simulink model "ABS_CAN_MBD"  (R2024b)
settings: Solver=FixedStepAuto  StartTime=0.0  StopTime=15  FixedStep=0.01  RelTol=1e-3
undefined symbols (not defined in the file): canChannel, g, I, m, R, v0
libraries: canlib x3, canmsglib x2
settings Model: Creator=Stephen Kingston  LastModifiedBy=chinmay
settings SolverCC: AlgebraicLoopSolver=TrustRegion
settings DebuggingCC: UnconnectedInputMsg=warning  UnconnectedOutputMsg=warning  UnconnectedLineMsg=warning
settings ModelReferenceCC: EnableRefExpFcnMdlSchedulingChecks=on
settings SFSimCC: CustomCodeUndefinedFunction=UseInterfaceOnly
settings RTWCC: GPUComputeCapability=3.5

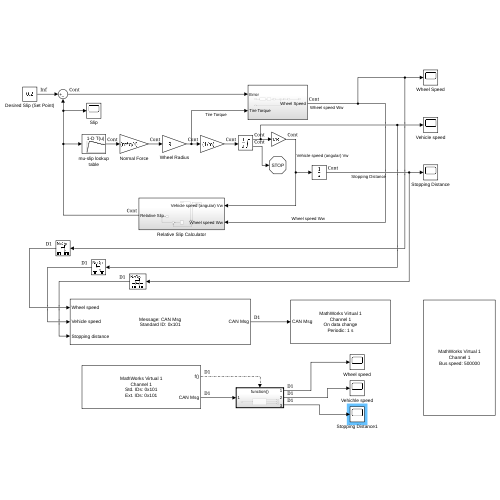
[thumbnail: Simulink's stored preview of the top-level diagram]
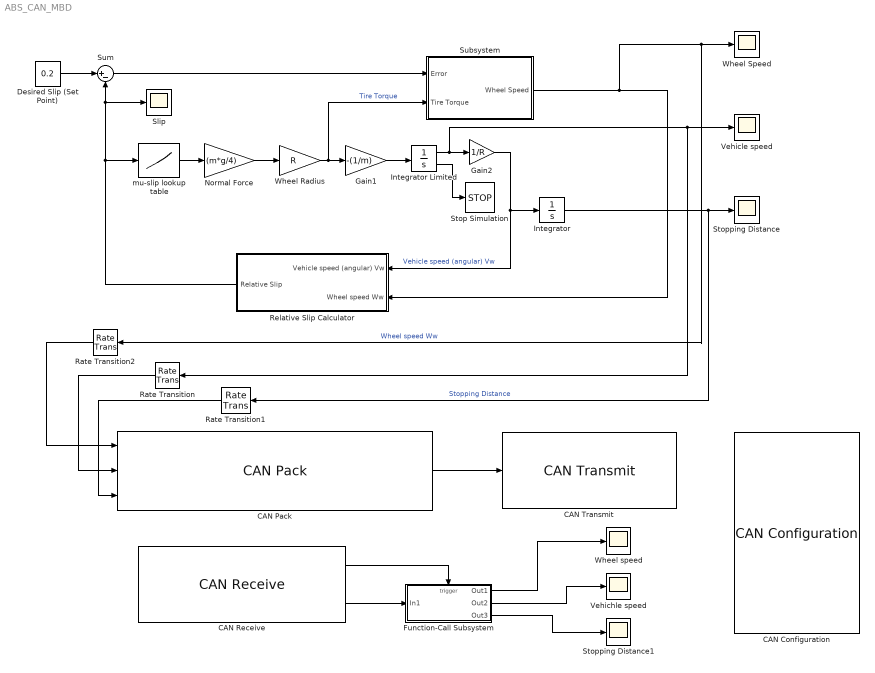
== system ABS_CAN_MBD ==
  CAN Configuration : canlib/CAN Configuration  BlockHandle=495.0005  Device=MathWorks Virtual 1 (Channel 1)  DeviceMenu=MathWorks Virtual 1 (Channel 1)  ObjConstructor=canChannel('MathWorks', 'Virtual 1', 1)  BusSpeed=500000  EnableBitParameters=off  AckMode=Normal
  CAN Pack : canmsglib/CAN Pack  MsgList=(none)  MsgName=CAN Msg  MsgIDType=Standard (11-bit identifier)  MsgIdentifier=0x101  CANIDInput=off  MsgLength=8  Remote=off  ApplyMinMax=off  BusOutput=off  SignalInfo={ 'Wheel speed', '0', '16', 'LE', 'unsigned', 'Standard', '0', '1', '0', '-Inf', 'Inf'; 'Vehicle speed', '16', '16', 'LE', 'unsigned', 'Standard', '0', '1', '0', '-Inf', 'Inf'; 'Stopping distance', '32', '16', 'LE', 'unsigned', 'Standard', '0', '1', '0', '-Inf', 'Inf' }
      settings: LibrarySourceBlock=canlib/CAN Pack  DataFormat=manually specified signals
  CAN Receive : canlib/CAN Receive  BlockHandle=500.0012  Device=MathWorks Virtual 1 (Channel 1)  DeviceMenu=MathWorks Virtual 1 (Channel 1)  ObjConstructor=canChannel('MathWorks', 'Virtual 1', 1)  EnableStandardIDsFilter=off  StdIDsCombo=Allow only  StandardIDs=0x101  EnableExtendedIDsFilter=off  ExtIDsCombo=Allow only  ExtendedIDs=0x101  SampleTime=0.01  MsgsPerTimestep=all  InternalFilterUpdateStatus=on  BusOutput=off
  CAN Transmit : canlib/CAN Transmit  BlockHandle=504.0006  Device=MathWorks Virtual 1 (Channel 1)  DeviceMenu=MathWorks Virtual 1 (Channel 1)  ObjConstructor=canChannel('MathWorks', 'Virtual 1', 1)  EnableEventTransmit=on  EnablePeriodicTransmit=on  MessagePeriod=1.000
  "Desired Slip (Set Point) " : Constant  Value=0.2
  Function-Call Subsystem : Subsystem  TreatAsAtomicUnit=on
  Gain1 : Gain  Gain=-(1/m)
  Gain2 : Gain  Gain=1/R
  Integrator : Integrator
  Integrator Limited : Integrator  InitialCondition=v0  LimitOutput=on  UpperSaturationLimit=1000  LowerSaturationLimit=0  ShowSaturationPort=on
  Normal Force : Gain  Gain=(m*g/4)
  Rate Transition : RateTransition  OutPortSampleTime=0.01
  Rate Transition1 : RateTransition  OutPortSampleTime=0.01
  Rate Transition2 : RateTransition  OutPortSampleTime=0.01
  Relative Slip Calculator : Subsystem
  "Slip " : Scope
  Stop Simulation : Stop
  Stopping Distance : Scope
  Stopping Distance1 : Scope
  Subsystem : Subsystem
  Sum : Sum  Inputs=|+-
  Vehichle speed : Scope
  Vehicle speed : Scope
  Wheel Radius : Gain  Gain=R
  Wheel Speed : Scope
  Wheel speed : Scope
  mu-slip lookup table : Lookup_n-D  NumberOfTableDimensions=1  BreakpointsForDimension1=[0,0.05,0.1,0.15,0.2,0.25,0.3,0.35,0.4,0.45,0.5,0.55,0.60,0.65,0.70,0.75,0.80,0.85,0.90,0.95,1]  Table=[0,0.4,0.8,0.97,1,0.98,0.96,0.94,0.92,0.9,0.88,0.855,0.83,0.81,0.79,0.77,0.75,0.73,0.72,0.71,0.7]  InternalRulePriority=Speed  RndMeth=Simplest
  wires:
  Sum/1 -> Subsystem/1(Error)
  Wheel Radius/1 -> Gain1/1, Subsystem/2(Tire Torque)  "Tire Torque"
  Gain2/1 -> Relative Slip Calculator/1(Vehicle speed (angular) Vw), Integrator/1  "Vehicle speed (angular) Vw"
  "Desired Slip (Set Point) "/1 -> Sum/1
  mu-slip lookup table/1 -> Normal Force/1
  Normal Force/1 -> Wheel Radius/1
  Gain1/1 -> Integrator Limited/1
  Integrator Limited/1 -> Rate Transition/1, Vehicle speed/1, Gain2/1
  Integrator/1 -> Stopping Distance/1, Rate Transition1/1  "Stopping Distance"
  Integrator Limited/2 -> Stop Simulation/1
  Subsystem/1(Wheel Speed) -> Rate Transition2/1, Wheel Speed/1, Relative Slip Calculator/2(Wheel speed Ww)  "Wheel speed Ww"
  Relative Slip Calculator/1(Relative Slip) -> "Slip "/1, Sum/2, mu-slip lookup table/1
  CAN Pack/1 -> CAN Transmit/1
  CAN Receive/2 -> Function-Call Subsystem/1(In1)
  CAN Receive/1 -> Function-Call Subsystem/Trigger
  Function-Call Subsystem/1(Out1) -> Wheel speed/1
  Function-Call Subsystem/2(Out2) -> Vehichle speed/1
  Function-Call Subsystem/3(Out3) -> Stopping Distance1/1
  Rate Transition2/1 -> CAN Pack/1
  Rate Transition/1 -> CAN Pack/2
  Rate Transition1/1 -> CAN Pack/3

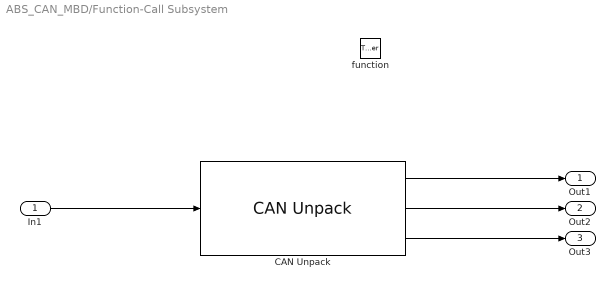
== system ABS_CAN_MBD/Function-Call Subsystem ==
  In1 : Inport
  function : TriggerPort  TriggerType=function-call  VariantControl=(inherit)
  CAN Unpack : canmsglib/CAN Unpack  MsgList=(none)  MsgName=CAN Msg  MsgIDType=Standard (11-bit identifier)  MsgIdentifier=0x101  MsgLength=8  SignalInfo={ 'Wheel speed', '0', '16', 'LE', 'unsigned', 'Standard', '0', '1', '0', '-Inf', 'Inf'; 'Vehicle speed', '16', '16', 'LE', 'unsigned', 'Standard', '0', '1', '0', '-Inf', 'Inf'; 'Stopping Distance', '32', '16', 'LE', 'unsigned', 'Standard', '0', '1', '0', '-Inf', 'Inf' }  IDPort=off  TimestampPort=off  ErrorPort=off  RemotePort=off  LengthPort=off  StatusPort=off  ApplyMinMax=off
      settings: LibrarySourceBlock=canlib/CAN Unpack
  Out1 : Outport
  Out2 : Outport  Port=2
  Out3 : Outport  Port=3
  wires:
  In1/1 -> CAN Unpack/1
  CAN Unpack/1 -> Out1/1
  CAN Unpack/3 -> Out3/1
  CAN Unpack/2 -> Out2/1

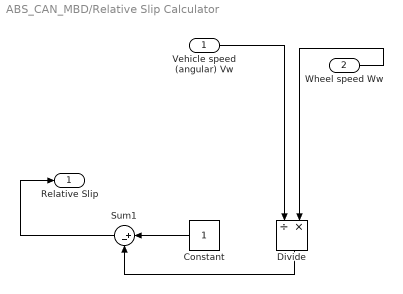
== system ABS_CAN_MBD/Relative Slip Calculator ==
  Vehicle speed (angular) Vw : Inport
  Wheel speed Ww : Inport  Port=2
  Constant : Constant
  Divide : Product  Inputs=/*
  Sum1 : Sum  Inputs=|+-
  Relative Slip : Outport  VectorParamsAs1DForOutWhenUnconnected=off
  wires:
  Divide/1 -> Sum1/2
  Sum1/1 -> Relative Slip/1
  Constant/1 -> Sum1/1
  Wheel speed Ww/1 -> Divide/2
  Vehicle speed (angular) Vw/1 -> Divide/1

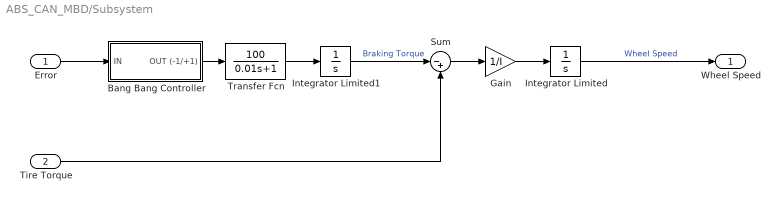
== system ABS_CAN_MBD/Subsystem ==
  Error : Inport
  Tire Torque : Inport  Port=2
  Bang Bang Controller : Subsystem
  Gain : Gain  Gain=1/I
  Integrator Limited : Integrator  InitialCondition=v0/R  LimitOutput=on  UpperSaturationLimit=1000  LowerSaturationLimit=0
  Integrator Limited1 : Integrator  LimitOutput=on  UpperSaturationLimit=1500  LowerSaturationLimit=0
  Sum : Sum  Inputs=|-+
  Transfer Fcn : TransferFcn  Numerator=[100]  Denominator=[0.01 1]
  Wheel Speed : Outport  VectorParamsAs1DForOutWhenUnconnected=off
  wires:
  Sum/1 -> Gain/1
  Transfer Fcn/1 -> Integrator Limited1/1
  Gain/1 -> Integrator Limited/1
  Integrator Limited/1 -> Wheel Speed/1  "Wheel Speed"
  Integrator Limited1/1 -> Sum/1  "Braking Torque"
  Bang Bang Controller/1(OUT (-1/+1)) -> Transfer Fcn/1
  Tire Torque/1 -> Sum/2
  Error/1 -> Bang Bang Controller/1(IN)

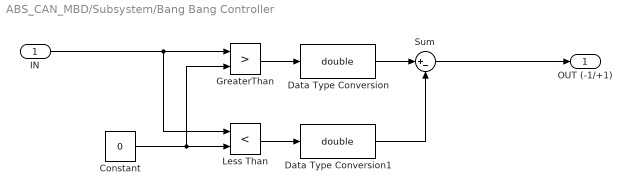
== system ABS_CAN_MBD/Subsystem/Bang Bang Controller ==
  IN : Inport
  Constant : Constant  Value=0
  Data Type Conversion : DataTypeConversion  OutDataTypeStr=double  SaturateOnIntegerOverflow=off
  Data Type Conversion1 : DataTypeConversion  OutDataTypeStr=double  SaturateOnIntegerOverflow=off
  GreaterThan : RelationalOperator  Operator=>  OutDataTypeStr=boolean  RndMeth=Simplest  InputSameDT=off
  Less Than : RelationalOperator  Operator=<  OutDataTypeStr=boolean  RndMeth=Simplest  InputSameDT=off
  Sum : Sum  Inputs=|+-
  OUT (-1/+1) : Outport  VectorParamsAs1DForOutWhenUnconnected=off
  wires:
  Sum/1 -> OUT (-1/+1)/1
  Data Type Conversion/1 -> Sum/1
  Constant/1 -> GreaterThan/2, Less Than/2
  IN/1 -> Less Than/1, GreaterThan/1
  Data Type Conversion1/1 -> Sum/2
  GreaterThan/1 -> Data Type Conversion/1
  Less Than/1 -> Data Type Conversion1/1
